simulink model "seEntityPriority"  (R2023b)
settings: Solver=VariableStepAuto  StartTime=0.0  StopTime=100  RelTol=1e-3  EnableMultiTasking=on
StopFcn:
  | hFig = sePlotPrioritizedDepartures(logsout);
undefined symbols (not defined in the file or in its folder): m
CloseFcn:
  | if exist('hFig')
  |     close(hFig);
  | end
  | clear logsout hFig
settings Model: Creator=The MathWorks, Inc.  LastModifiedBy=alfre
settings SolverCC: AlgebraicLoopSolver=TrustRegion
settings DataIOCC: SaveOutput=off  DSMLogging=off  SaveTime=off  ReturnWorkspaceOutputs=off
settings OptimizationCC: LifeSpan=inf
settings DebuggingCC: UnconnectedInputMsg=warning  UnconnectedOutputMsg=warning  UnconnectedLineMsg=warning  SFUnexpectedBacktrackingDiag=warning  SFNoUnconditionalDefaultTransitionDiag=warning  SFExecutionAtInitializationDiag=none  ArithmeticOperatorsInVariantConditions=warning
settings ModelReferenceCC: EnableRefExpFcnMdlSchedulingChecks=on
settings SFSimCC: SimUseLocalCustomCode=off  CustomCodeUndefinedFunction=UseInterfaceOnly
settings RTWCC: RTWUseLocalCustomCode=off  DLArmComputeVersion=19.05
settings CodeAppCC: StateflowObjectComments=on
settings GRTTargetCC: TargetLangStandard=C89/C90 (ANSI)
settings ConfigComp: CovMetricSettings=dw  CovSaveCumulativeToWorkspaceVar=on  CovSaveSingleToWorkspaceVar=on  CovExternalEMLEnable=off

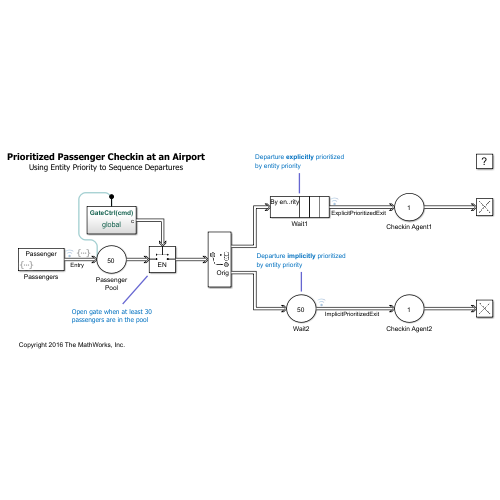
[thumbnail: Simulink's stored preview of the top-level diagram]
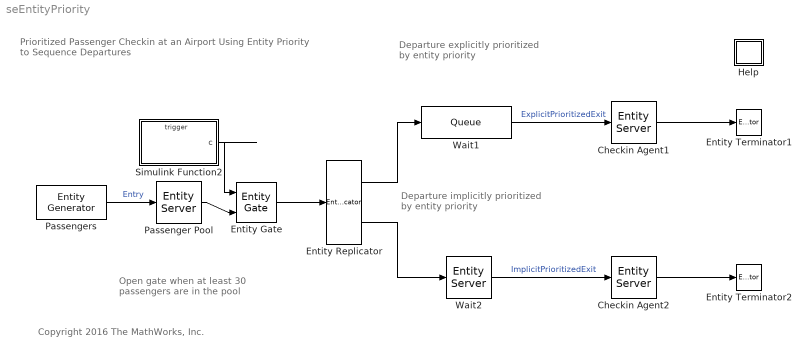
== system seEntityPriority ==
  note: Copyright 2016 The MathWorks, Inc.
  note: Prioritized Passenger Checkin at an Airport
      | Using Entity Priority to Sequence Departures
  note: Open gate when at least 30
      | passengers are in the pool
  note: Departure explicitly prioritized
      | by entity priority
  note: Departure implicitly prioritized
      | by entity priority
  Checkin Agent1 : EntityServer  InputPortMessageModes=m  OutputPortMessageModes=m  Capacity=1  ServiceTimeSource=Attribute  ServiceTimeAttributeName=CheckinTime
  Checkin Agent2 : EntityServer  InputPortMessageModes=m  OutputPortMessageModes=m  Capacity=1  ServiceTimeSource=Attribute  ServiceTimeAttributeName=CheckinTime
  Entity Gate : EntityGate  InputPortMessageModes=m,m  OutputPortMessageModes=m
  Entity Replicator : EntityReplicator  InputPortMessageModes=m  OutputPortMessageModes=m,m  HoldOriginalEntityUntilAllReplicasDepart=on
  Entity Terminator1 : EntityTerminator  InputPortMessageModes=m
  Entity Terminator2 : EntityTerminator  InputPortMessageModes=m
  Help : Subsystem
      settings: OpenFcn=showExample('simevents/EntityPriorityExample');
      mask Display: disp('?')
  Passenger Pool : EntityServer  InputPortMessageModes=m  OutputPortMessageModes=m  Capacity=50  ServiceTimeValue=0  ServiceTimeAttributeName=CheckinTime  EntryAction=|
      | persistent nEntered
      | if isempty(nEntered)
      |     nEntered = 0;
      | end
      | 
      | nEntered = nEntered + 1;
      | 
      | if nEntered == 30
      |     GateCtrl(1);
      | end
  Passengers : EntityGenerator  OutputPortMessageModes=m  TimeSource=MATLAB action  IntergenerationTimeAction=|  GenerateAction=|  AttributeName=Class|CheckinTime  AttributeInitialValue=1|0  EntityType=Structured  EntityTypeName=Passenger  EntityPriority=1
      IntergenerationTimeAction=|
      | persistent entCount 
      | if isempty(entCount)
      |     entCount = 0;
      | end
      | if entCount == 29
      |     dt = inf;
      | else
      |     dt = 0;
      | end
      | 
      | entCount = entCount + 1;
      GenerateAction=|
      | persistent entCount
      | if isempty(entCount)
      |     entCount = 1;
      | end
      | 
      | %entity.Class = 3-ceil(entCount/10)+1;
      | entity.Class = randi(3);
      | entity.CheckinTime = rand()+1;
      | entitySys.priority = entity.Class;
      | 
      | entCount = entCount + 1;
  Simulink Function2 : Subsystem  TreatAsAtomicUnit=on
  Wait1 : Queue  InputPortMessageModes=m  OutputPortMessageModes=m  Capacity=50  QueueType=Priority  PrioritySource=entitySys.priority
  Wait2 : EntityServer  InputPortMessageModes=m  OutputPortMessageModes=m  Capacity=50  ServiceTimeValue=0  ServiceTimeAttributeName=CheckinTime
  wires:
  Wait1/1 -> Checkin Agent1/1  "ExplicitPrioritizedExit"
  Checkin Agent1/1 -> Entity Terminator1/1
  Checkin Agent2/1 -> Entity Terminator2/1
  Wait2/1 -> Checkin Agent2/1  "ImplicitPrioritizedExit"
  Entity Replicator/2 -> Wait2/1
  Entity Replicator/1 -> Wait1/1
  Passengers/1 -> Passenger Pool/1  "Entry"
  Entity Gate/1 -> Entity Replicator/1
  Simulink Function2/1(c) -> Entity Gate/1
  Passenger Pool/1 -> Entity Gate/2

== system seEntityPriority/Help ==

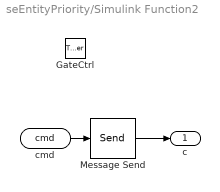
== system seEntityPriority/Simulink Function2 ==
  GateCtrl : TriggerPort  TriggerType=function-call  IsSimulinkFunction=on  FunctionName=GateCtrl  VariantControl=Variant
  Message Send : Send  OutputPortMessageModes=m
  cmd : ArgIn  ArgumentName=cmd
  c : Outport
  wires:
  cmd/1 -> Message Send/1
  Message Send/1 -> c/1
